simulink model "Glider_Simulink"  (R2019a)
settings: Solver=VariableStepAuto  StartTime=0.0  StopTime=10.0  RelTol=1e-3
values from neighbouring files (symbols this model uses):
  alpha_0 = -2.5 * (pi/(180))    (= -0.0436332312999)    [Glider_Sim.m]
  AR = 11.08    [Glider_Sim.m]
  Cd_0 = 0.01    [Glider_Sim.m]
  CD_E = 0.002    [Glider_Sim.m]
  CD_F = 0.008    [Glider_Sim.m]
  Cd_L = 0.05    [Glider_Sim.m]
  CD_T = 0.01    [Glider_Sim.m]
  CL_alpha = (a_0)/(1+(a_0)/(pi*e*AR))    (= 4.88344983796)    [Glider_Sim.m]
  CL_min = 0.4    [Glider_Sim.m]
  e = 0.95    [Glider_Sim.m]
  S = (l^2)/(AR)    (= 946.368231047)    [Glider_Sim.m]
  S_F = 216    [Glider_Sim.m]
  S_T = (V_H*c_bar*S)/(l_t)    (= 125.678091539)    [Glider_Sim.m]
  S_V = (V_V*l*S)/(l_t)    (= 67.5977307891)    [Glider_Sim.m]
libraries: simulink x1
settings Model: Creator=Wian  LastModifiedBy=Wian

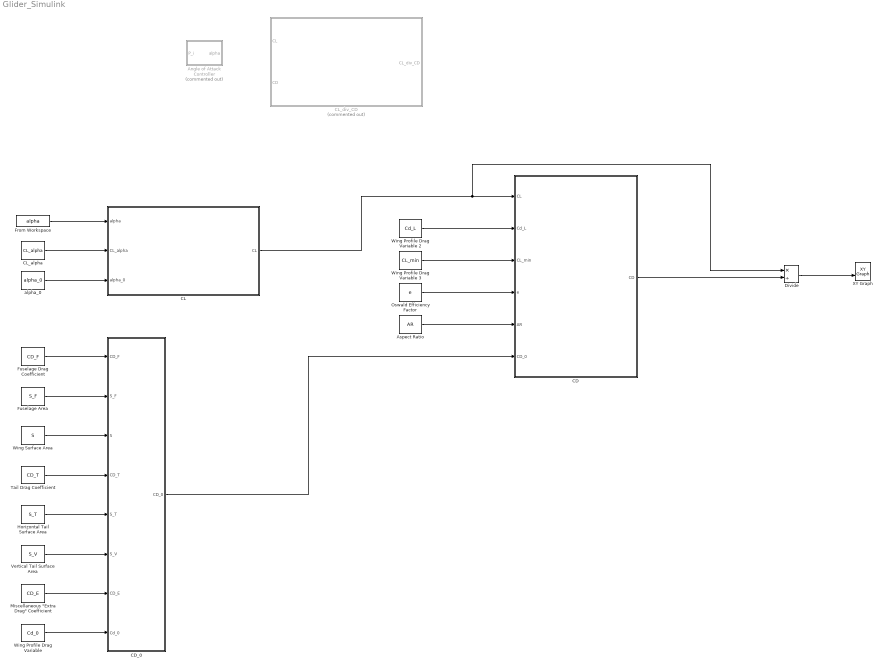
== system Glider_Simulink ==
  Angle of Attack Controller : MATLAB Function  Commented=on  TreatAsAtomicUnit=on
  Aspect Ratio : Constant  Value=AR
  CD : MATLAB Function  TreatAsAtomicUnit=on
  CD_0 : MATLAB Function  TreatAsAtomicUnit=on
  CL : MATLAB Function  TreatAsAtomicUnit=on
  CL_alpha : Constant  Value=CL_alpha
  CL_div_CD : MATLAB Function  Commented=on  TreatAsAtomicUnit=on
  Divide : Product  Inputs=*/
  From Workspace : FromWorkspace  VariableName=alpha  SampleTime=0
  Fuselage Area : Constant  Value=S_F
  Fuselage Drag Coefficient : Constant  Value=CD_F
  Horizontal Tail Surface Area : Constant  Value=S_T
  "Miscellaneous \"Extra Drag\" Coefficient" : Constant  Value=CD_E
  Oswald Efficiency Factor : Constant  Value=e
  Tail Drag Coefficient : Constant  Value=CD_T
  Vertical Tail Surface Area : Constant  Value=S_V
  Wing Profile Drag Variable : Constant  Value=Cd_0
  Wing Profile Drag Variable 2 : Constant  Value=Cd_L
  "Wing Profile Drag Variable 3 " : Constant  Value=CL_min
  "Wing Surface Area " : Constant  Value=S
  XY Graph : simulink/Sinks/XY Graph  xmin=-1  xmax=1  ymin=-1  ymax=1  st=-1
  alpha_0 : Constant  Value=alpha_0
  wires:
  alpha_0/1 -> CL/3(alpha_0)
  CL_alpha/1 -> CL/2(CL_alpha)
  CL/1(CL) -> Divide/1, CD/1(CL)
  CD_0/1(CD_0) -> CD/6(CD_0)
  Fuselage Drag Coefficient/1 -> CD_0/1(CD_F)
  Fuselage Area/1 -> CD_0/2(S_F)
  "Wing Surface Area "/1 -> CD_0/3(S)
  Tail Drag Coefficient/1 -> CD_0/4(CD_T)
  Horizontal Tail Surface Area/1 -> CD_0/5(S_T)
  Vertical Tail Surface Area/1 -> CD_0/6(S_V)
  "Miscellaneous \"Extra Drag\" Coefficient"/1 -> CD_0/7(CD_E)
  Wing Profile Drag Variable/1 -> CD_0/8(Cd_0)
  Aspect Ratio/1 -> CD/5(AR)
  Oswald Efficiency Factor/1 -> CD/4(e)
  "Wing Profile Drag Variable 3 "/1 -> CD/3(CL_min)
  Wing Profile Drag Variable 2/1 -> CD/2(Cd_L)
  From Workspace/1 -> CL/1(alpha)
  CD/1(CD) -> Divide/2
  Divide/1 -> XY Graph/2

== matlab function Glider_Simulink/CL ==
  data: alpha input; CL output; CL_alpha input; alpha_0 input
% Lift Coefficient which is a function of alpha
function CL = CL_calc(alpha, CL_alpha, alpha_0)
    CL = CL_alpha*(alpha - alpha_0);  
end

== matlab function Glider_Simulink/Angle of Attack Controller ==
  data: P_i input; alpha output
function alpha = fcn(P_i)
% function alpha = fcn(P_i)
% This function calculates the new angle of attack (alpha) iteratively in order to
% re-orient dynamically and vertically the aircraft trajectory towards the
% target position. 
% 
% function alpha = fcn(P_i)   %TODO Add bank angle variable as well
% 
% syms alpha
% 
% 
% % Lift Coefficient function of alpha
% CL = CL_alpha*(alpha - alpha_0);        
% 
% % Drag Coefficient function of alpha
% CD = CD_0 + Cd_L*(CL - CL_min)^2 + ((CL)^2)/(pi*e*AR);
% 
% % Tangent of the angle between the direction vector P_i to the target point. 
% Gi_numerator = P_i(3);
% 
% Gi_denominator = sqrt(((P_i(1))^2) -((P_i(2))^2));
% 
% Gi = (Gi_numerator)/(Gi_denominator);
% end

== matlab function Glider_Simulink/CD ==
  data: CL input; Cd_L input; CL_min input; e input; AR input; CD_0 input; CD output
% Drag Coefficient which is a function of alpha
function CD = CD_calc(CL,Cd_L,CL_min,e,AR,CD_0)
    CD = CD_0 + Cd_L*(CL - CL_min).^2 + (CL.^2)/(pi*e*AR); 
end

== matlab function Glider_Simulink/CD_0 ==
  data: CD_F input; CD_0 output; S_F input; S input; CD_T input; S_T input; S_V input; CD_E input; Cd_0 input
% Constant Part of Total Drag Formula
function CD_0 = CD_0_calc(CD_F,S_F,S,CD_T,S_T,S_V,CD_E,Cd_0)
    CD_0 = (CD_F*S_F)/(S) + (CD_T*(S_T + S_V))/(S) + CD_E + Cd_0;  

end

== matlab function Glider_Simulink/CL_div_CD ==
  data: CL input; CL_div_CD output; CD input
% Plot CL/CD
function CL_div_CD = CL_div_CD(CL,CD)
   CL_div_CD = (CL)/(CD);
end
